simulink model "dotproduct_test"  (Simulink 8.7)
settings: Solver=ode45  StartTime=0.0  StopTime=10.0  RelTol=1e-3
settings Model: Creator=arnaud  LastModifiedBy=hamza
settings DataIOCC: SaveFormat=Structure
settings DebuggingCC: UnderspecifiedInitializationDetection=Simplified  MergeDetectMultiDrivingBlocksExec=error  SolverPrmCheckMsg=warning
settings ConfigComp: CovSFcnEnable=off

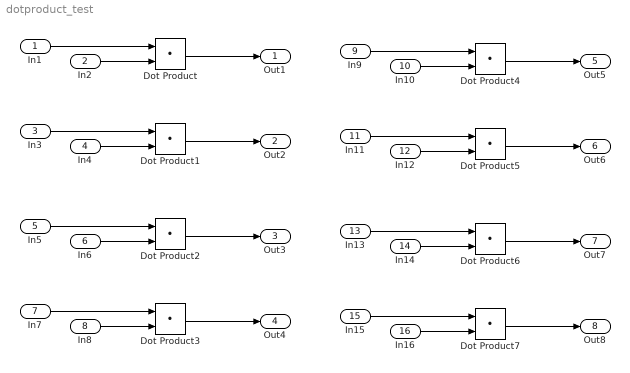
== system dotproduct_test ==
  In1 : Inport  OutDataTypeStr=int8  PortDimensions=3
      settings: SignalType=complex
  In2 : Inport  Port=2  OutDataTypeStr=int8  PortDimensions=[1 3]
  In3 : Inport  Port=3  OutDataTypeStr=double  PortDimensions=3
  In4 : Inport  Port=4  OutDataTypeStr=double  PortDimensions=[1 3]
      settings: SignalType=complex
  In5 : Inport  Port=5  OutDataTypeStr=int8  PortDimensions=1
      settings: SignalType=complex
  In6 : Inport  Port=6  OutDataTypeStr=int8  PortDimensions=1
  In7 : Inport  Port=7  OutDataTypeStr=double  PortDimensions=1
  In8 : Inport  Port=8  OutDataTypeStr=double  PortDimensions=1
      settings: SignalType=complex
  In9 : Inport  Port=9  OutDataTypeStr=int8  PortDimensions=1
      settings: SignalType=complex
  In10 : Inport  Port=10  OutDataTypeStr=int8  PortDimensions=1
      settings: SignalType=complex
  In11 : Inport  Port=11  OutDataTypeStr=double  PortDimensions=1
      settings: SignalType=complex
  In12 : Inport  Port=12  OutDataTypeStr=double  PortDimensions=1
      settings: SignalType=complex
  In13 : Inport  Port=13  OutDataTypeStr=double  PortDimensions=1
  In14 : Inport  Port=14  OutDataTypeStr=double  PortDimensions=1
  In15 : Inport  Port=15  OutDataTypeStr=double  PortDimensions=3
  In16 : Inport  Port=16  OutDataTypeStr=double  PortDimensions=[1 3]
  Dot Product{,1..7} (8 alike) : DotProduct  InputSameDT=on  OutDataTypeStr=Inherit: Inherit via internal rule
  Out1 : Outport
  Out2 : Outport  Port=2
  Out3 : Outport  Port=3
  Out4 : Outport  Port=4
  Out5 : Outport  Port=5
  Out6 : Outport  Port=6
  Out7 : Outport  Port=7
  Out8 : Outport  Port=8
  wires:
  In2/1 -> Dot Product/2
  In1/1 -> Dot Product/1
  Dot Product/1 -> Out1/1
  In4/1 -> Dot Product1/2
  Dot Product1/1 -> Out2/1
  In3/1 -> Dot Product1/1
  In6/1 -> Dot Product2/2
  In5/1 -> Dot Product2/1
  Dot Product2/1 -> Out3/1
  In8/1 -> Dot Product3/2
  Dot Product3/1 -> Out4/1
  In7/1 -> Dot Product3/1
  In10/1 -> Dot Product4/2
  In9/1 -> Dot Product4/1
  Dot Product4/1 -> Out5/1
  In12/1 -> Dot Product5/2
  Dot Product5/1 -> Out6/1
  In11/1 -> Dot Product5/1
  In14/1 -> Dot Product6/2
  Dot Product6/1 -> Out7/1
  In13/1 -> Dot Product6/1
  In16/1 -> Dot Product7/2
  Dot Product7/1 -> Out8/1
  In15/1 -> Dot Product7/1
